simulink model "M009_refor_control_SOFC"  (R2021a)
settings: Solver=ode23tb  StartTime=0.0  StopTime=0.011794  RelTol=1e-3
undefined symbols (not defined in the file): MM_vec, nearst_p, p, Target, TotalMassTarget, Tr, Ts, x0_SOFC
libraries: pid_lib x1
settings Model: Creator=djoroya  LastModifiedBy=djoroya

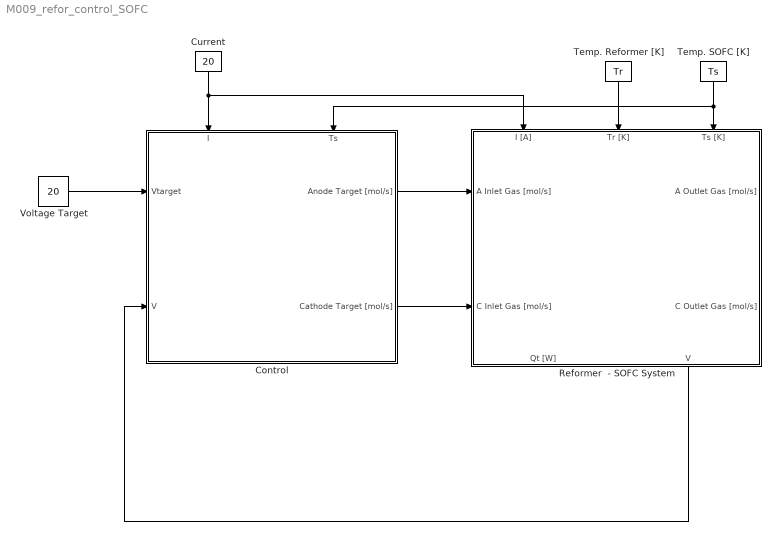
== system M009_refor_control_SOFC ==
  Control : Subsystem
      settings: PortSchema="{\"entries\":[{\"content\":{\"sides\":[{\"content\":{\"connectorIds\":[\"In1\",\"In2\"]},\"type\":\"ConnectorPlacement.EquallySpacedRectSide\",\"uuid\":\"b973b84c-8793-4046-ac9f-d89f915fcc30\"},{\"content\":{\"connectorIds\":[\"Out1\",\"Out2\"],\"side\":\"RIGHT\"},\"type\":\"ConnectorPlacement.EquallySpacedRectSide\",\"uuid\":\"99065125-60e5-4151-bf81-1bc55728c1bd\"},{\"content\":{\"connectorIds\":[\"In3\",\"In4\"],\"side\":\"TOP\"},\"type\":\"ConnectorPlacement.EquallySpacedRectSide\",\"uuid\":\"8b4e6a96-1b8a-4203-9bc5-ee7dbc8914e0\"}]},\"type\":\"ConnectorPlacement.EquallySpacedConnector\",\"uuid\":\"b75553d6-16dc-45b9-a76a-e219211962db\"}],\"packageUris\":[\"http://schema.mathworks.com/mf0/Connector/R2020b\"],\"version\":\"1.0\"}"
  Current : Constant  Value=20
  Reformer  - SOFC System : Subsystem
      settings: PortSchema="{\"entries\":[{\"content\":{\"sides\":[{\"content\":{\"connectorIds\":[\"In1\",\"In2\"]},\"type\":\"ConnectorPlacement.EquallySpacedRectSide\",\"uuid\":\"200e76d3-d0bd-400d-80aa-1287817324e9\"},{\"content\":{\"connectorIds\":[\"Out1\",\"Out2\"],\"side\":\"RIGHT\"},\"type\":\"ConnectorPlacement.EquallySpacedRectSide\",\"uuid\":\"3a1b6d1c-88bc-44b4-af37-27ac9ade1ff0\"},{\"content\":{\"connectorIds\":[\"In3\",\"In4\",\"In5\"],\"side\":\"TOP\"},\"type\":\"ConnectorPlacement.EquallySpacedRectSide\",\"uuid\":\"7d8c75f4-d537-4a2f-8caa-a1e3e4142219\"},{\"content\":{\"connectorIds\":[\"Out3\",\"Out4\"],\"side\":\"BOTTOM\"},\"type\":\"ConnectorPlacement.EquallySpacedRectSide\",\"uuid\":\"773ed184-9145-4e58-8690-ed7d817bf4e6\"}]},\"type\":\"ConnectorPlacement.EquallySpacedConnector\",\"uuid\":\"9e56a9e7-d63f-4491-bdfd-789be4cca736\"}],\"packageUris\":[\"http://schema.mathworks.com/mf0/Connector/R2020b\"],\"version\":\"1.0\"}"
  Temp. Reformer [K] : Constant  Value=Tr
  Temp. SOFC [K] : Constant  Value=Ts
  Voltage Target : Constant  Value=20
  wires:
  Control/1(Anode Target [mol/s]) -> Reformer  - SOFC System/1(A Inlet Gas [mol/s])
  Temp. Reformer [K]/1 -> Reformer  - SOFC System/4(Tr [K])
  Temp. SOFC [K]/1 -> Control/4(Ts), Reformer  - SOFC System/5(Ts [K])
  Control/2("Cathode Target [mol/s] ") -> Reformer  - SOFC System/2(C Inlet Gas [mol/s])
  Current/1 -> Reformer  - SOFC System/3(I [A]), Control/3(I)
  Voltage Target/1 -> Control/1(Vtarget)
  Reformer  - SOFC System/4(V) -> Control/2(V)

== system M009_refor_control_SOFC/Control ==
  Vtarget : Inport
  V : Inport  Port=2
  I : Inport  Port=3
  Ts : Inport  Port=4
  From Workspace : FromWorkspace  VariableName=air_mol_inlet_flow
  Product : Product
  Scope : Scope
  Target : Constant  Value=TotalMassTarget
  Target1 : Constant  Value=Target
  Anode Target [mol/s] : Outport
  "Cathode Target [mol/s] " : Outport  Port=2
  wires:
  From Workspace/1 -> "Cathode Target [mol/s] "/1
  Target/1 -> Product/2
  Product/1 -> Scope/1, Anode Target [mol/s]/1
  Target1/1 -> Product/1

== system M009_refor_control_SOFC/Reformer  - SOFC System ==
  note: Fuel
      | A node
      | (H2,O2,H2O,N2,CO,CH4,CO2,Diesel,Ar,Csoot)
      | [mol/s]
  A Inlet Gas [mol/s] : Inport
  C Inlet Gas [mol/s] : Inport  Port=2
  I [A] : Inport  Port=3
  Tr [K] : Inport  Port=4
  Ts [K] : Inport  Port=5
  Minus : Sum  Inputs=+-
  Product1 : Product
  Reformer Controlled : Subsystem
      settings: PortSchema="{\"entries\":[{\"content\":{\"sides\":[{\"content\":{\"connectorIds\":[\"In1\"]},\"type\":\"ConnectorPlacement.EquallySpacedRectSide\",\"uuid\":\"29baeb98-2fcd-4e93-bac7-89db238943a7\"},{\"content\":{\"connectorIds\":[\"Out1\"],\"side\":\"RIGHT\"},\"type\":\"ConnectorPlacement.EquallySpacedRectSide\",\"uuid\":\"d0aab1a2-46f5-4965-965a-81b00350cf0c\"},{\"content\":{\"connectorIds\":[\"In2\"],\"side\":\"TOP\"},\"type\":\"ConnectorPlacement.EquallySpacedRectSide\",\"uuid\":\"1acf7f26-ad42-41c1-b7e9-1e1e0c97fb8d\"}]},\"type\":\"ConnectorPlacement.EquallySpacedConnector\",\"uuid\":\"b24af2ad-4c30-4b70-9d7f-38f68bce100c\"}],\"packageUris\":[\"http://schema.mathworks.com/mf0/Connector/R2020b\"],\"version\":\"1.0\"}"
  SOFC Cell : Subsystem  mask{p=p, x0=x0_SOFC}
      mask prompts: p "params"
      settings: PortSchema="{\"entries\":[{\"content\":{\"sides\":[{\"content\":{\"connectorIds\":[\"In1\",\"In2\",\"In3\"]},\"type\":\"ConnectorPlacement.EquallySpacedRectSide\",\"uuid\":\"6cca8e4f-6db2-48de-a60a-b6fbc16877c6\"},{\"content\":{\"connectorIds\":[\"Out1\",\"Out2\",\"Out3\",\"Out4\"],\"side\":\"RIGHT\"},\"type\":\"ConnectorPlacement.EquallySpacedRectSide\",\"uuid\":\"c481f6d1-531d-4215-9ae0-5807376c0625\"},{\"content\":{\"connectorIds\":[\"In4\"],\"side\":\"TOP\"},\"type\":\"ConnectorPlacement.EquallySpacedRectSide\",\"uuid\":\"76720726-927e-4340-b17d-e33f4db2c782\"},{\"content\":{\"connectorIds\":[\"Out5\",\"Out6\"],\"side\":\"BOTTOM\"},\"type\":\"ConnectorPlacement.EquallySpacedRectSide\",\"uuid\":\"7ed108e3-6588-44d6-8f3d-9789ffe258a7\"}]},\"type\":\"ConnectorPlacement.EquallySpacedConnector\",\"uuid\":\"f9228f26-0840-43d6-932a-2fdb8a27bf20\"}],\"packageUris\":[\"http://schema.mathworks.com/mf0/Connector/R2020b\"],\"version\":\"1.0\"}"
  A Outlet Gas [mol/s] : Outport
  C Outlet Gas [mol/s] : Outport  Port=2
  Qt [W] : Outport  Port=3
  V : Outport  Port=4
  wires:
  A Inlet Gas [mol/s]/1 -> Reformer Controlled/1(Target MolarFlow [mol/s])
  SOFC Cell/5(EThermal) -> Minus/1  "ET"
  SOFC Cell/3(vc) -> C Outlet Gas [mol/s]/1  "pc_out [mol/s]"
  I [A]/1 -> SOFC Cell/2(I), Product1/2  "I"
  C Inlet Gas [mol/s]/1 -> SOFC Cell/3(Air[mol/s])
  SOFC Cell/6(Voltaje) -> Minus/2, V/1  "V"
  SOFC Cell/2(va) -> A Outlet Gas [mol/s]/1  "pa_out [mol/s]"
  Reformer Controlled/1(Actual Molar Flow [mol/s]) -> SOFC Cell/1(qin_anode)  "qin_anode"
  Product1/1 -> Qt [W]/1
  Minus/1 -> Product1/1
  Tr [K]/1 -> Reformer Controlled/2(T)
  Ts [K]/1 -> SOFC Cell/4(T)

== system M009_refor_control_SOFC/Reformer  - SOFC System/Reformer Controlled ==
  Target MolarFlow [mol/s] : Inport
  T : Inport  Port=2
  "Controler " : Subsystem
      settings: PortSchema="{\"entries\":[{\"content\":{\"sides\":[{\"content\":{\"connectorIds\":[\"In1\",\"In2\"]},\"type\":\"ConnectorPlacement.EquallySpacedRectSide\",\"uuid\":\"d0df8d63-6ccb-4e17-b5ac-849eda0159c4\"},{\"content\":{\"connectorIds\":[\"Out1\",\"Out2\",\"Out3\"],\"side\":\"RIGHT\"},\"type\":\"ConnectorPlacement.EquallySpacedRectSide\",\"uuid\":\"810d19ce-f80f-4df6-8135-9424920dd639\"},{\"content\":{\"connectorIds\":[],\"side\":\"TOP\"},\"type\":\"ConnectorPlacement.EquallySpacedRectSide\",\"uuid\":\"28b6769f-9191-4787-8749-9b059fcc021d\"},{\"content\":{\"connectorIds\":[\"In3\"],\"side\":\"BOTTOM\"},\"type\":\"ConnectorPlacement.EquallySpacedRectSide\",\"uuid\":\"5627e3a9-abda-41c8-96fd-097f9bf3cc2c\"}]},\"type\":\"ConnectorPlacement.EquallySpacedConnector\",\"uuid\":\"98d8d06d-7f78-4370-9651-63955ba4785e\"}],\"packageUris\":[\"http://schema.mathworks.com/mf0/Connector/R2020b\"],\"version\":\"1.0\"}"
  Gain : Gain  Gain=1./MM_vec
  Gain1 : Gain  Gain=MM_vec
  "Reformer " : Subsystem
  Actual Molar Flow [mol/s] : Outport
  wires:
  Gain/1 -> Actual Molar Flow [mol/s]/1  "out"
  Target MolarFlow [mol/s]/1 -> Gain1/1
  "Controler "/3(Steam) -> "Reformer "/3(Steam)  "Steam"
  "Controler "/2(Air) -> "Reformer "/2(Air)  "Air"
  "Controler "/1(Diesel) -> "Reformer "/1(Diesel)  "Diesel"
  Gain1/1 -> "Controler "/2(Target)
  T/1 -> "Controler "/3(T), "Reformer "/4(T)
  "Reformer "/1(MassFlows) -> "Controler "/1(MassFlow), Gain/1

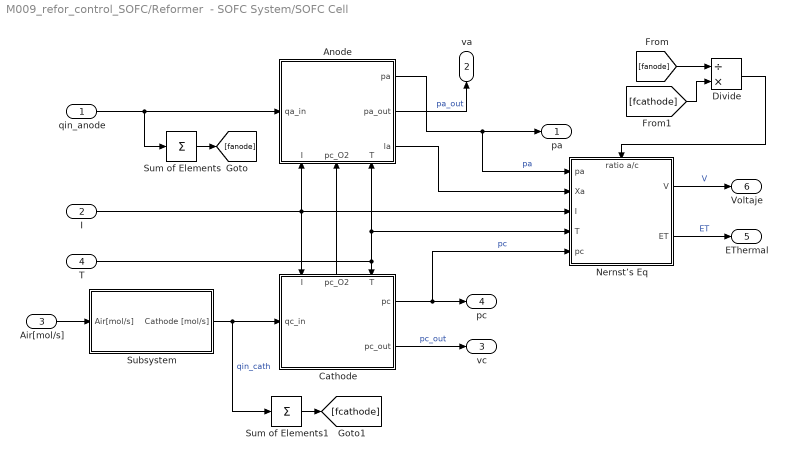
== system M009_refor_control_SOFC/Reformer  - SOFC System/SOFC Cell ==
  qin_anode : Inport
  I : Inport  Port=2
  Air[mol/s] : Inport  Port=3
  T : Inport  Port=4
  Anode : Subsystem
      settings: PortSchema="{\"entries\":[{\"content\":{\"sides\":[{\"content\":{\"connectorIds\":[\"In1\"]},\"type\":\"ConnectorPlacement.EquallySpacedRectSide\",\"uuid\":\"1d27f661-9cb9-482d-ac43-89e84d52643b\"},{\"content\":{\"connectorIds\":[\"Out1\",\"Out2\",\"Out3\"],\"side\":\"RIGHT\"},\"type\":\"ConnectorPlacement.EquallySpacedRectSide\",\"uuid\":\"62ac897d-5819-4e9c-a19f-e210851aefa2\"},{\"content\":{\"connectorIds\":[],\"side\":\"TOP\"},\"type\":\"ConnectorPlacement.EquallySpacedRectSide\",\"uuid\":\"1380e9d4-c5ac-42ce-b6fc-00336cc8edba\"},{\"content\":{\"connectorIds\":[\"In2\",\"In3\",\"In4\"],\"side\":\"BOTTOM\"},\"type\":\"ConnectorPlacement.EquallySpacedRectSide\",\"uuid\":\"0e36fd1a-38eb-48cb-8834-06d558b43614\"}]},\"type\":\"ConnectorPlacement.EquallySpacedConnector\",\"uuid\":\"79a72313-dbdc-4de5-b88f-787bafe984c7\"}],\"packageUris\":[\"http://schema.mathworks.com/mf0/Connector/R2020b\"],\"version\":\"1.0\"}"
  Cathode : Subsystem
      settings: PortSchema="{\"entries\":[{\"content\":{\"sides\":[{\"content\":{\"connectorIds\":[\"In1\"]},\"type\":\"ConnectorPlacement.EquallySpacedRectSide\",\"uuid\":\"1d27f661-9cb9-482d-ac43-89e84d52643b\"},{\"content\":{\"connectorIds\":[\"Out1\",\"Out2\"],\"side\":\"RIGHT\"},\"type\":\"ConnectorPlacement.EquallySpacedRectSide\",\"uuid\":\"62ac897d-5819-4e9c-a19f-e210851aefa2\"},{\"content\":{\"connectorIds\":[\"In2\",\"Out3\",\"In3\"],\"side\":\"TOP\"},\"type\":\"ConnectorPlacement.EquallySpacedRectSide\",\"uuid\":\"1380e9d4-c5ac-42ce-b6fc-00336cc8edba\"}]},\"type\":\"ConnectorPlacement.EquallySpacedConnector\",\"uuid\":\"79a72313-dbdc-4de5-b88f-787bafe984c7\"}],\"packageUris\":[\"http://schema.mathworks.com/mf0/Connector/R2020b\"],\"version\":\"1.0\"}"
  Divide : Product  Inputs=/*
  "Nernst’s Eq " : Subsystem
      settings: PortSchema="{\"entries\":[{\"content\":{\"sides\":[{\"content\":{\"connectorIds\":[\"In1\",\"In2\",\"In3\",\"In4\",\"In5\"]},\"type\":\"ConnectorPlacement.EquallySpacedRectSide\",\"uuid\":\"1b300774-e64d-4a8a-a2e9-ecdc71723fee\"},{\"content\":{\"connectorIds\":[\"Out1\",\"Out2\"],\"side\":\"RIGHT\"},\"type\":\"ConnectorPlacement.EquallySpacedRectSide\",\"uuid\":\"354a04f1-cc66-4a63-8c50-8080316e29e9\"},{\"content\":{\"connectorIds\":[\"In6\"],\"side\":\"TOP\"},\"type\":\"ConnectorPlacement.EquallySpacedRectSide\",\"uuid\":\"b48b7bda-dd37-468f-ab7d-ccd563a69f0b\"}]},\"type\":\"ConnectorPlacement.EquallySpacedConnector\",\"uuid\":\"ddfd4041-6e53-4893-9028-34e5ff9f82d6\"}],\"packageUris\":[\"http://schema.mathworks.com/mf0/Connector/R2020b\"],\"version\":\"1.0\"}"
  Subsystem : Subsystem
  Sum of Elements : Sum  Inputs=+
  Sum of Elements1 : Sum  Inputs=+
  pa : Outport
  va : Outport  Port=2
  vc : Outport  Port=3
  pc : Outport  Port=4
  EThermal : Outport  Port=5
  Voltaje : Outport  Port=6
  wires:
  Air[mol/s]/1 -> Subsystem/1(Air[mol/s])
  Anode/1(pa) -> pa/1, "Nernst’s Eq "/1(pa)  "pa"
  Anode/2(pa_out) -> va/1  "pa_out"
  Cathode/1(pc) -> "Nernst’s Eq "/5(pc), pc/1  "pc"
  Subsystem/1(Cathode [mol/s]) -> Sum of Elements1/1, Cathode/1(qc_in)  "qin_cath"
  "Nernst’s Eq "/2(ET) -> EThermal/1  "ET"
  Cathode/3(pc_O2) -> Anode/3(pc_O2)
  Cathode/2(pc_out) -> vc/1  "pc_out"
  I/1 -> Cathode/2(I), "Nernst’s Eq "/3(I), Anode/2(I)
  T/1 -> "Nernst’s Eq "/4(T), Anode/4(T), Cathode/3(T)
  qin_anode/1 -> Anode/1(qa_in), Sum of Elements/1
  "Nernst’s Eq "/1(V) -> Voltaje/1  "V"
  Anode/3(la) -> "Nernst’s Eq "/2(Xa)
  Sum of Elements/1 -> [fanode]
  Sum of Elements1/1 -> [fcathode]
  [fanode] -> Divide/1
  [fcathode] -> Divide/2
  Divide/1 -> "Nernst’s Eq "/6(ratio a/c)

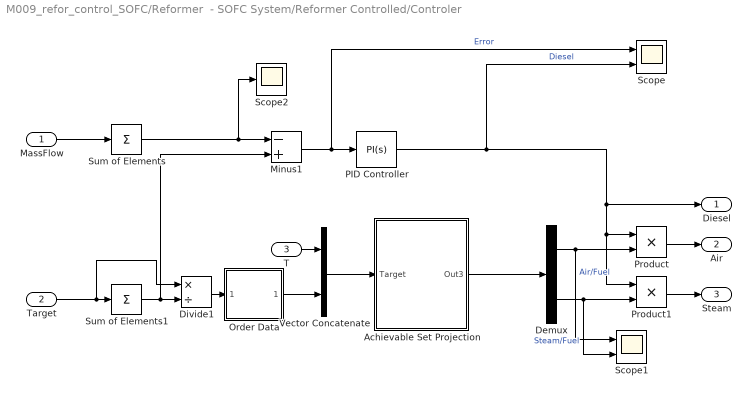
== system M009_refor_control_SOFC/Reformer  - SOFC System/Reformer Controlled/Controler  ==
  MassFlow : Inport
  Target : Inport  Port=2
  T : Inport  Port=3
  Achievable Set Projection : Subsystem
  Demux : Demux  Outputs=2
  Divide1 : Product  Inputs=*/
  Minus1 : Sum  Inputs=-+
  Order Data : Subsystem
  PID Controller : pid_lib/PID Controller  Controller=PI  Form=Parallel  TimeDomain=Continuous-time  UseExternalTs=off  SampleTime=-1  IntegratorMethod=Forward Euler  FilterMethod=Forward Euler  ControllerParametersSource=internal  P=10  I=50  D=1  UseFilter=on  N=100  TunerSelectOption=Transfer Function Based (PID Tuner App)  ZeroCross=off  InitialConditionSource=internal  InitialConditionForIntegrator=0  InitialConditionForFilter=0  DifferentiatorICPrevScaledInput=0  ExternalReset=none  TrackingMode=off  Kt=1  LimitOutput=off  SatLimitsSource=internal  UpperSaturationLimit=inf  LowerSaturationLimit=-inf  LinearizeAsGain=on  AntiWindupMode=none  Kb=1  POutMin=[]  POutMax=[]  IOutMin=[]  IOutMax=[]  DOutMin=[]  DOutMax=[]  NOutMin=[]  NOutMax=[]  SumOutMin=[]  SumOutMax=[]  SaturationOutMin=[]  SaturationOutMax=[]  PParamMin=[]  PParamMax=[]  IParamMin=[]  IParamMax=[]  DParamMin=[]  DParamMax=[]  NParamMin=[]  NParamMax=[]  KbParamMin=[]  KbParamMax=[]  KtParamMin=[]  KtParamMax=[]  KbOutMin=[]  KbOutMax=[]  KtOutMin=[]  KtOutMax=[]  IntegratorOutMin=[]  IntegratorOutMax=[]  FilterOutMin=[]  FilterOutMax=[]  SumI1OutMin=[]  SumI1OutMax=[]  SumI2OutMin=[]  SumI2OutMax=[]  SumI3OutMin=[]  SumI3OutMax=[]  SumI4OutMin=[]  SumI4OutMax=[]  SumDOutMin=[]  SumDOutMax=[]  DifferentiatorOutMin=[]  DifferentiatorOutMax=[]  FilterDiffOutCoefMin=[]  FilterDiffOutCoefMax=[]  ReciprocalOutMin=[]  ReciprocalOutMax=[]  SumDenOutMin=[]  SumDenOutMax=[]  SumNumOutMin=[]  SumNumOutMax=[]  DivideOutMin=[]  DivideOutMax=[]  UdiffTsProdOutMin=[]  UdiffTsProdOutMax=[]  NTsProdOutMin=[]  NTsProdOutMax=[]  UintegralTsProdOutMin=[]  UintegralTsProdOutMax=[]  UngainTsProdOutMin=[]  UngainTsProdOutMax=[]  IntegratorContinuousStateAttributes=''  IntegratorStateMustResolveToSignalObject=off  IntegratorRTWStateStorageClass=Auto  FilterContinuousStateAttributes=''  FilterStateMustResolveToSignalObject=off  FilterRTWStateStorageClass=Auto  ParallelPVariant=InternalParameters  IdealPVariant=Disabled  IVariant=InternalParameters  DVariant=Disabled  IntegratorVariant=Continuous  SatVariant=Disabled  AWVariant=Passthrough  PCopyVariant=Disabled  TRVariant=Disabled  FdbkBlocksVariant=Forward  IdealPFdbkVariant=Disabled  SatFdbkVariant=Disabled  DerivativeFilterVariant=Disabled  NVariant=Disabled  NCopyVariant=Disabled_SignalSpec  FilterICVariant=Disabled  IntegratorICVariant=InternalICs  ExternalResetVariant=Disabled  TRSumVariant=Passthrough  SumFdbkVariant=Disabled  SumVariant=Sum_PI  TsampFilterVariant=InternalTs  TsampNgainVariant=Passthrough  TsampIntegralVariant=Passthrough  ExternalSaturationOutDataTypeStr=Inherit: Same as second input
  Product : Product
  Product1 : Product
  Scope : Scope  NumInputPorts=2
  Scope1 : Scope  NumInputPorts=2
  Scope2 : Scope
  Sum of Elements : Sum  Inputs=+
  Sum of Elements1 : Sum  Inputs=+
  Vector Concatenate : Concatenate
  Diesel : Outport
  Air : Outport  Port=2
  Steam : Outport  Port=3
  wires:
  Product/1 -> Air/1
  Demux/1 -> Scope1/1, Product/2  "Air/Fuel"
  Demux/2 -> Scope1/2, Product1/2  "Steam/Fuel"
  Product1/1 -> Steam/1
  Sum of Elements/1 -> Scope2/1, Minus1/1
  T/1 -> Vector Concatenate/1
  Order Data/1(Out1) -> Vector Concatenate/2
  Sum of Elements1/1 -> Divide1/2, Minus1/2
  Target/1 -> Divide1/1, Sum of Elements1/1
  Divide1/1 -> Order Data/1(Target)
  Minus1/1 -> PID Controller/1, Scope/1  "Error"
  MassFlow/1 -> Sum of Elements/1
  PID Controller/1 -> Product1/1, Product/1, Diesel/1, Scope/2  "Diesel"
  Vector Concatenate/1 -> Achievable Set Projection/1(Target)
  Achievable Set Projection/1(Out3) -> Demux/1

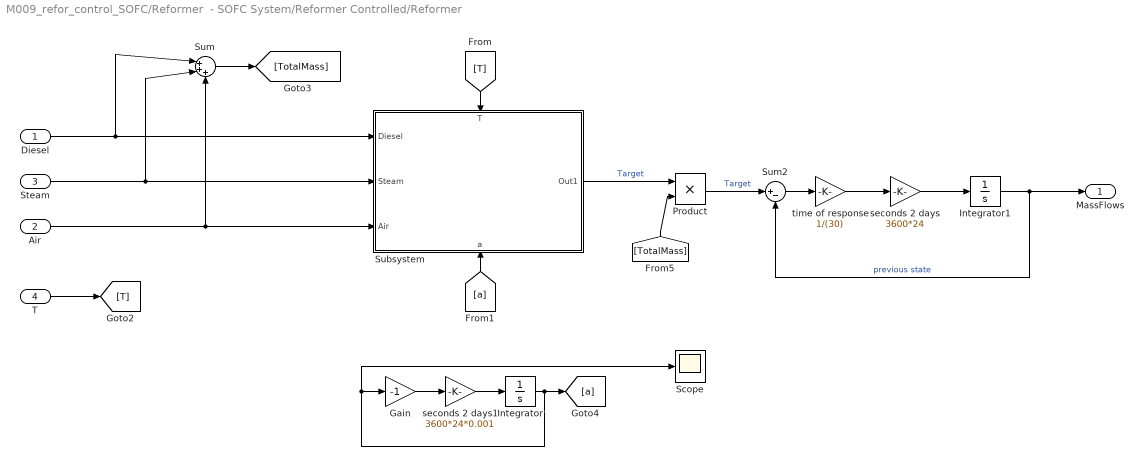
== system M009_refor_control_SOFC/Reformer  - SOFC System/Reformer Controlled/Reformer  ==
  Diesel : Inport
  Air : Inport  Port=2
  Steam : Inport  Port=3
  T : Inport  Port=4
  Gain : Gain  Gain=-1
  Integrator : Integrator  InitialCondition=1
  Integrator1 : Integrator  InitialCondition=1e-6
  Product : Product
  Scope : Scope
  Subsystem : Subsystem
      settings: PortSchema="{\"entries\":[{\"content\":{\"sides\":[{\"content\":{\"connectorIds\":[\"In1\",\"In2\",\"In3\"]},\"type\":\"ConnectorPlacement.EquallySpacedRectSide\",\"uuid\":\"0dada652-6957-4c3e-8e48-73ee360a3bab\"},{\"content\":{\"connectorIds\":[\"Out1\"],\"side\":\"RIGHT\"},\"type\":\"ConnectorPlacement.EquallySpacedRectSide\",\"uuid\":\"81208621-951c-43f9-b655-3502a16ce57a\"},{\"content\":{\"connectorIds\":[\"In4\"],\"side\":\"TOP\"},\"type\":\"ConnectorPlacement.EquallySpacedRectSide\",\"uuid\":\"1012e2be-7d0b-44a9-9a40-bc453950010e\"},{\"content\":{\"connectorIds\":[\"In5\"],\"side\":\"BOTTOM\"},\"type\":\"ConnectorPlacement.EquallySpacedRectSide\",\"uuid\":\"aaef83a2-abb7-4780-82b5-9abad57d39ad\"}]},\"type\":\"ConnectorPlacement.EquallySpacedConnector\",\"uuid\":\"1143871f-aacc-4fa7-a444-9910d5016eff\"}],\"packageUris\":[\"http://schema.mathworks.com/mf0/Connector/R2020b\"],\"version\":\"1.0\"}"
  Sum : Sum  Inputs=|+++
  Sum2 : Sum  Inputs=|+-
  seconds 2 days : Gain  Gain=3600*24
  seconds 2 days1 : Gain  Gain=3600*24*0.001
  time of response : Gain  Gain=1/(30)
  MassFlows : Outport
  wires:
  T/1 -> [T]
  Sum/1 -> [TotalMass]
  [TotalMass] -> Product/2
  Diesel/1 -> Sum/1, Subsystem/1(Diesel)
  seconds 2 days1/1 -> Integrator/1
  Gain/1 -> seconds 2 days1/1
  [a] -> Subsystem/5(a)
  [T] -> Subsystem/4(T)
  time of response/1 -> seconds 2 days/1
  Sum2/1 -> time of response/1
  Product/1 -> Sum2/1  "Target"
  seconds 2 days/1 -> Integrator1/1
  Integrator1/1 -> MassFlows/1, Sum2/2  "previous state"
  Subsystem/1(Out1) -> Product/1  "Target"
  Steam/1 -> Sum/2, Subsystem/2(Steam)
  Air/1 -> Sum/3, Subsystem/3(Air)
  Integrator/1 -> Scope/1, Gain/1, [a]

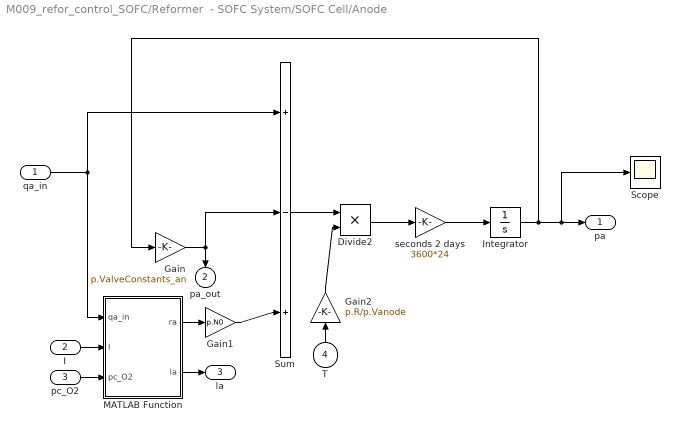
== system M009_refor_control_SOFC/Reformer  - SOFC System/SOFC Cell/Anode ==
  qa_in : Inport
  I : Inport  Port=2
  pc_O2 : Inport  Port=3
  T : Inport  Port=4
  Divide2 : Product  Inputs=**
  Gain : Gain  Gain=p.ValveConstants_an
  Gain1 : Gain  Gain=p.N0
  Gain2 : Gain  Gain=p.R/p.Vanode
  Integrator : Integrator  InitialCondition=x0_SOFC.pa
  MATLAB Function : MATLAB Function  TreatAsAtomicUnit=on
  Scope : Scope
  Sum : Sum  Inputs=|+-+
  seconds 2 days : Gain  Gain=3600*24
  pa : Outport
  pa_out : Outport  Port=2
  la : Outport  Port=3
  wires:
  Sum/1 -> Divide2/1
  Integrator/1 -> Scope/1, pa/1, Gain/1
  Gain2/1 -> Divide2/2
  qa_in/1 -> Sum/1, MATLAB Function/1(qa_in)
  Gain/1 -> pa_out/1, Sum/2
  I/1 -> MATLAB Function/2(I)
  T/1 -> Gain2/1
  MATLAB Function/2(la) -> la/1
  pc_O2/1 -> MATLAB Function/3(pc_O2)
  MATLAB Function/1(ra) -> Gain1/1
  Gain1/1 -> Sum/3
  Divide2/1 -> seconds 2 days/1
  seconds 2 days/1 -> Integrator/1

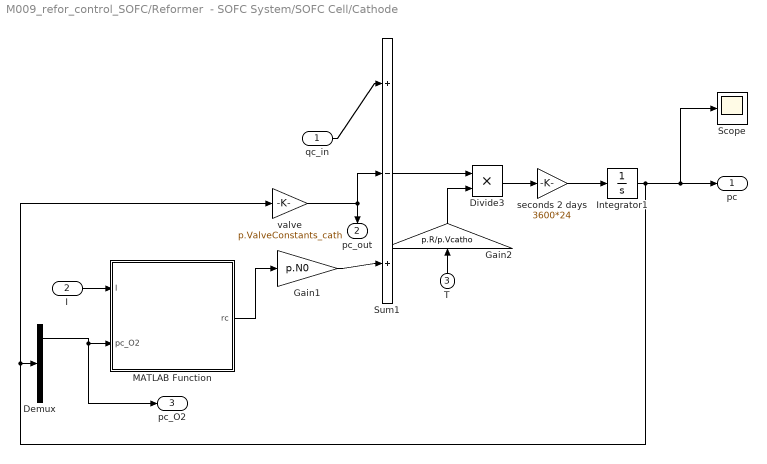
== system M009_refor_control_SOFC/Reformer  - SOFC System/SOFC Cell/Cathode ==
  qc_in : Inport
  I : Inport  Port=2
  T : Inport  Port=3
  Demux : Demux  Outputs=8
  Divide3 : Product  Inputs=**
  Gain1 : Gain  Gain=p.N0
  Gain2 : Gain  Gain=p.R/p.Vcatho
  Integrator1 : Integrator  InitialCondition=x0_SOFC.pc
  MATLAB Function : MATLAB Function  TreatAsAtomicUnit=on
  Scope : Scope
  Sum1 : Sum  Inputs=|+-+
  seconds 2 days : Gain  Gain=3600*24
  valve : Gain  Gain=p.ValveConstants_cath
  pc : Outport
  pc_out : Outport  Port=2  Unit=mol/s
  pc_O2 : Outport  Port=3
  wires:
  Sum1/1 -> Divide3/1
  Integrator1/1 -> valve/1, Demux/1, Scope/1, pc/1
  qc_in/1 -> Sum1/1
  Gain2/1 -> Divide3/2
  T/1 -> Gain2/1
  valve/1 -> pc_out/1, Sum1/2
  I/1 -> MATLAB Function/1(I)
  Demux/2 -> pc_O2/1, MATLAB Function/2(pc_O2)
  MATLAB Function/1(rc) -> Gain1/1
  Gain1/1 -> Sum1/3
  Divide3/1 -> seconds 2 days/1
  seconds 2 days/1 -> Integrator1/1

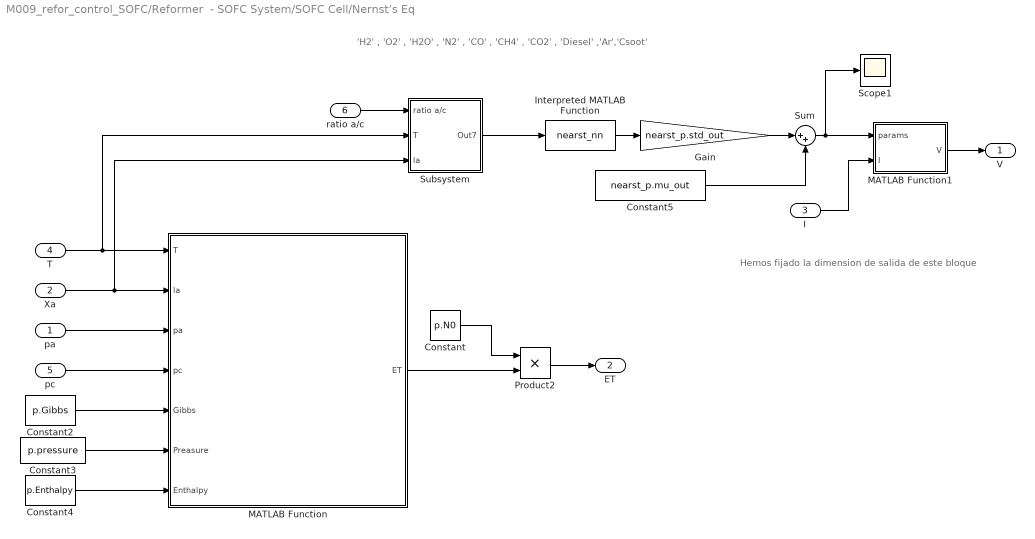
== system M009_refor_control_SOFC/Reformer  - SOFC System/SOFC Cell/Nernst’s Eq  ==
  note: Hemos fijado la dimension de salida de este bloque
  note: 'H2' , 'O2' , 'H2O' , 'N2' , 'CO' , 'CH4' , 'CO2' , 'Diesel' ,'Ar','Csoot'
  pa : Inport
  Xa : Inport  Port=2
  I : Inport  Port=3
  T : Inport  Port=4
  pc : Inport  Port=5
  ratio a/c : Inport  Port=6
  Constant : Constant  Value=p.N0
  Constant2 : Constant  Value=p.Gibbs  OutDataTypeStr=Bus:slBus1
  Constant3 : Constant  Value=p.pressure
  Constant4 : Constant  Value=p.Enthalpy  OutDataTypeStr=Bus:slBus1
  Constant5 : Constant  Value=nearst_p.mu_out
  Gain : Gain  Gain=nearst_p.std_out
  Interpreted MATLAB Function : MATLABFcn  MATLABFcn=nearst_nn
  MATLAB Function : MATLAB Function  TreatAsAtomicUnit=on
  MATLAB Function1 : MATLAB Function  TreatAsAtomicUnit=on
  Product2 : Product
  Scope1 : Scope
  Subsystem : Subsystem
  Sum : Sum  Inputs=|++
  V : Outport  PortDimensions=1
  ET : Outport  Port=2  PortDimensions=1
  wires:
  pa/1 -> MATLAB Function/3(pa)
  pc/1 -> MATLAB Function/4(pc)
  Constant2/1 -> MATLAB Function/5(Gibbs)
  T/1 -> MATLAB Function/1(T), Subsystem/2(T)
  Xa/1 -> MATLAB Function/2(la), Subsystem/3(la)
  Constant3/1 -> MATLAB Function/6(Preasure)
  Constant4/1 -> MATLAB Function/7(Enthalpy)
  Product2/1 -> ET/1
  MATLAB Function/1(ET) -> Product2/2
  ratio a/c/1 -> Subsystem/1(ratio a/c)
  Subsystem/1(Out7) -> Interpreted MATLAB Function/1
  Interpreted MATLAB Function/1 -> Gain/1
  Gain/1 -> Sum/1
  Constant5/1 -> Sum/2
  Sum/1 -> Scope1/1, MATLAB Function1/1(params)
  MATLAB Function1/1(V) -> V/1
  Constant/1 -> Product2/1
  I/1 -> MATLAB Function1/2(I)

== system M009_refor_control_SOFC/Reformer  - SOFC System/SOFC Cell/Subsystem ==
  Air[mol/s] : Inport
  Molar Fractions (H2,O2,H2O,N2,CO,CH4,CO2) [mol/(Air-mol)] : Constant  Value=[0 0.2095 0 0.7808 0 0 0 0 0 0]
  Product : Product
  Cathode [mol/s] : Outport
  wires:
  Air[mol/s]/1 -> Product/1  "Air [mol/s]"
  Product/1 -> Cathode [mol/s]/1  "Cathode [mol/s]"
  Molar Fractions (H2,O2,H2O,N2,CO,CH4,CO2) [mol/(Air-mol)]/1 -> Product/2

== system M009_refor_control_SOFC/Reformer  - SOFC System/Reformer Controlled/Controler /Achievable Set Projection ==
  Target : Inport
  Abs : Abs
  Equilibrium2Ratios : MATLABFcn  MATLABFcn=backward_reformer_net  OutputDimensions=2  OutputSignalType=real  Output1D=off
  If : If  IfExpression=u1 > 0.01
  If Action Subsystem : Subsystem  TreatAsAtomicUnit=on
  If Action Subsystem1 : Subsystem  TreatAsAtomicUnit=on
  Merge : Merge
  ¿Convex hull? : MATLABFcn  MATLABFcn=check_convex_hull  OutputDimensions=1  OutputSignalType=real  Output1D=off
  Out3 : Outport
  wires:
  ¿Convex hull?/1 -> If/1
  Target/1 -> If Action Subsystem1/1(Target), If Action Subsystem/1(Target), ¿Convex hull?/1
  If/1 -> If Action Subsystem/Action
  If/2 -> If Action Subsystem1/Action
  Merge/1 -> Equilibrium2Ratios/1
  If Action Subsystem/1(Out1) -> Merge/1
  If Action Subsystem1/1(Out1) -> Merge/2
  Equilibrium2Ratios/1 -> Abs/1
  Abs/1 -> Out3/1

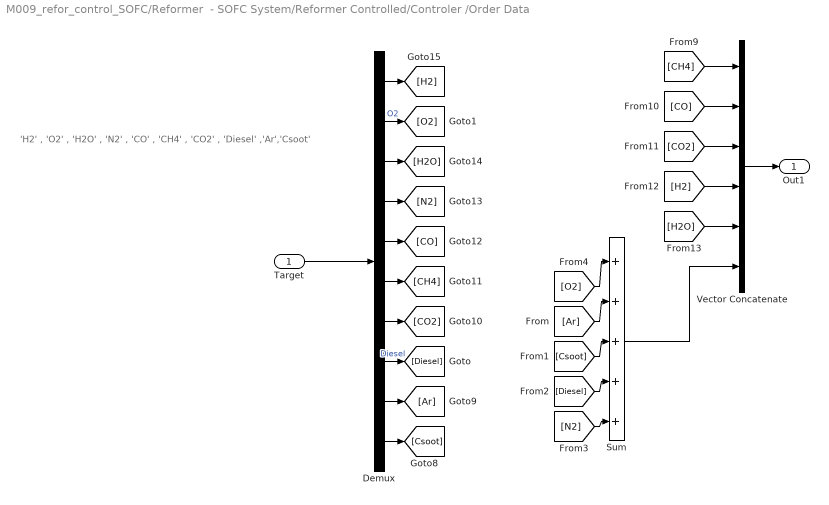
== system M009_refor_control_SOFC/Reformer  - SOFC System/Reformer Controlled/Controler /Order Data ==
  note: 'H2' , 'O2' , 'H2O' , 'N2' , 'CO' , 'CH4' , 'CO2' , 'Diesel' ,'Ar','Csoot'
  Target : Inport
  Demux : Demux  Outputs=10
  Sum : Sum  Inputs=|+++++
  Vector Concatenate : Concatenate  NumInputs=6
  Out1 : Outport
  wires:
  Target/1 -> Demux/1
  [CO] -> Vector Concatenate/2
  [CO2] -> Vector Concatenate/3
  [H2] -> Vector Concatenate/4
  [H2O] -> Vector Concatenate/5
  Vector Concatenate/1 -> Out1/1
  Demux/1 -> [H2]
  Demux/3 -> [H2O]
  Demux/4 -> [N2]
  Demux/5 -> [CO]
  Demux/6 -> [CH4]
  Demux/7 -> [CO2]
  Demux/9 -> [Ar]
  Demux/10 -> [Csoot]
  [CH4] -> Vector Concatenate/1
  Demux/2 -> [O2]  "O2"
  Demux/8 -> [Diesel]  "Diesel"
  [O2] -> Sum/1
  [Ar] -> Sum/2
  [Csoot] -> Sum/3
  [Diesel] -> Sum/4
  [N2] -> Sum/5
  Sum/1 -> Vector Concatenate/6

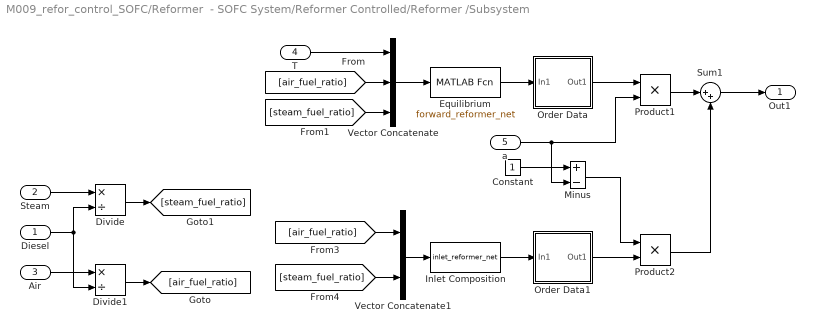
== system M009_refor_control_SOFC/Reformer  - SOFC System/Reformer Controlled/Reformer /Subsystem ==
  Diesel : Inport
  Steam : Inport  Port=2
  Air : Inport  Port=3
  T : Inport  Port=4
  a : Inport  Port=5
  Constant : Constant
  Divide : Product  Inputs=*/
  Divide1 : Product  Inputs=*/
  Equilibrium : MATLABFcn  MATLABFcn=forward_reformer_net  OutputDimensions=8  OutputSignalType=real  Output1D=off
  Inlet Composition : MATLABFcn  MATLABFcn=inlet_reformer_net  OutputDimensions=6  OutputSignalType=real  Output1D=off
  Minus : Sum  Inputs=+-
  Order Data : Subsystem
  Order Data1 : Subsystem
  Product1 : Product
  Product2 : Product
  Sum1 : Sum  Inputs=|++
  Vector Concatenate : Concatenate  NumInputs=3
  Vector Concatenate1 : Concatenate
  Out1 : Outport
  wires:
  a/1 -> Product1/2, Minus/2
  [steam_fuel_ratio] -> Vector Concatenate/3
  Product1/1 -> Sum1/1
  T/1 -> Vector Concatenate/1
  [air_fuel_ratio] -> Vector Concatenate1/1
  Vector Concatenate/1 -> Equilibrium/1
  Product2/1 -> Sum1/2
  [steam_fuel_ratio] -> Vector Concatenate1/2
  Order Data1/1(Out1) -> Product2/2
  Minus/1 -> Product2/1
  Inlet Composition/1 -> Order Data1/1(In1)
  Order Data/1(Out1) -> Product1/1
  Vector Concatenate1/1 -> Inlet Composition/1
  [air_fuel_ratio] -> Vector Concatenate/2
  Equilibrium/1 -> Order Data/1(In1)
  Constant/1 -> Minus/1
  Sum1/1 -> Out1/1
  Steam/1 -> Divide/1
  Diesel/1 -> Divide1/2, Divide/2
  Air/1 -> Divide1/1
  Divide/1 -> [steam_fuel_ratio]
  Divide1/1 -> [air_fuel_ratio]

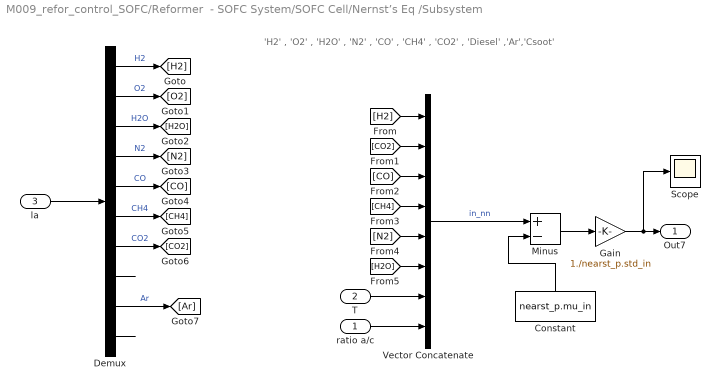
== system M009_refor_control_SOFC/Reformer  - SOFC System/SOFC Cell/Nernst’s Eq /Subsystem ==
  note: 'H2' , 'O2' , 'H2O' , 'N2' , 'CO' , 'CH4' , 'CO2' , 'Diesel' ,'Ar','Csoot'
  ratio a/c : Inport
  T : Inport  Port=2
  la : Inport  Port=3
  Constant : Constant  Value=nearst_p.mu_in
  Demux : Demux  Outputs=10
  Gain : Gain  Gain=1./nearst_p.std_in
  Minus : Sum  Inputs=+-
  Scope : Scope
  Vector Concatenate : Concatenate  NumInputs=8
  Out7 : Outport
  wires:
  Demux/7 -> [CO2]  "CO2"
  la/1 -> Demux/1
  Demux/3 -> [H2O]  "H2O"
  Demux/1 -> [H2]  "H2"
  Demux/8 -> ?
  Demux/2 -> [O2]  "O2"
  Demux/10 -> ?
  Demux/9 -> [Ar]  "Ar"
  Demux/5 -> [CO]  "CO"
  Demux/4 -> [N2]  "N2"
  Demux/6 -> [CH4]  "CH4"
  ratio a/c/1 -> Vector Concatenate/8
  T/1 -> Vector Concatenate/7
  [H2] -> Vector Concatenate/1
  [CO2] -> Vector Concatenate/2
  [CO] -> Vector Concatenate/3
  [CH4] -> Vector Concatenate/4
  [N2] -> Vector Concatenate/5
  [H2O] -> Vector Concatenate/6
  Vector Concatenate/1 -> Minus/1  "in_nn"
  Constant/1 -> Minus/2
  Minus/1 -> Gain/1
  Gain/1 -> Scope/1, Out7/1

== system M009_refor_control_SOFC/Reformer  - SOFC System/Reformer Controlled/Controler /Achievable Set Projection/If Action Subsystem ==
  Target : Inport
  Action Port : ActionPort  ActionPortLabel=if(u1 > 0.01)
  Demux : Demux  Outputs=7
  Vector Concatenate : Concatenate
  proyection : MATLABFcn  MATLABFcn=proyection_in_convex_hull  OutputDimensions=6  OutputSignalType=real  Output1D=off
  Out1 : Outport
  wires:
  Target/1 -> Demux/1, proyection/1
  proyection/1 -> Vector Concatenate/2
  Demux/1 -> Vector Concatenate/1
  Vector Concatenate/1 -> Out1/1

== system M009_refor_control_SOFC/Reformer  - SOFC System/Reformer Controlled/Controler /Achievable Set Projection/If Action Subsystem1 ==
  Target : Inport
  Action Port : ActionPort  ActionPortLabel=else
  Out1 : Outport
  wires:
  Target/1 -> Out1/1

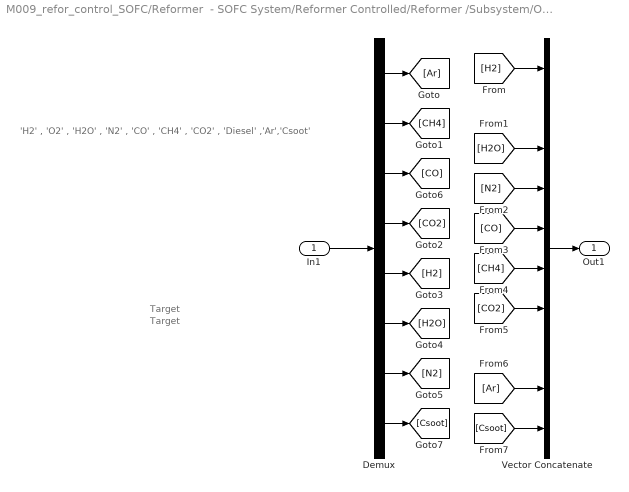
== system M009_refor_control_SOFC/Reformer  - SOFC System/Reformer Controlled/Reformer /Subsystem/Order Data ==
  note: Target
  note: Target
  note: 'H2' , 'O2' , 'H2O' , 'N2' , 'CO' , 'CH4' , 'CO2' , 'Diesel' ,'Ar','Csoot'
  In1 : Inport
  Demux : Demux  Outputs=8
  Vector Concatenate : Concatenate  NumInputs=10
  Out1 : Outport
  wires:
  In1/1 -> Demux/1
  Demux/1 -> [Ar]
  Demux/2 -> [CH4]
  Demux/3 -> [CO]
  Demux/4 -> [CO2]
  Demux/5 -> [H2]
  Demux/6 -> [H2O]
  Demux/7 -> [N2]
  Demux/8 -> [Csoot]
  [H2] -> Vector Concatenate/1
  [H2O] -> Vector Concatenate/3
  [N2] -> Vector Concatenate/4
  [CO] -> Vector Concatenate/5
  [CH4] -> Vector Concatenate/6
  [CO2] -> Vector Concatenate/7
  [Ar] -> Vector Concatenate/9
  [Csoot] -> Vector Concatenate/10
  Vector Concatenate/1 -> Out1/1

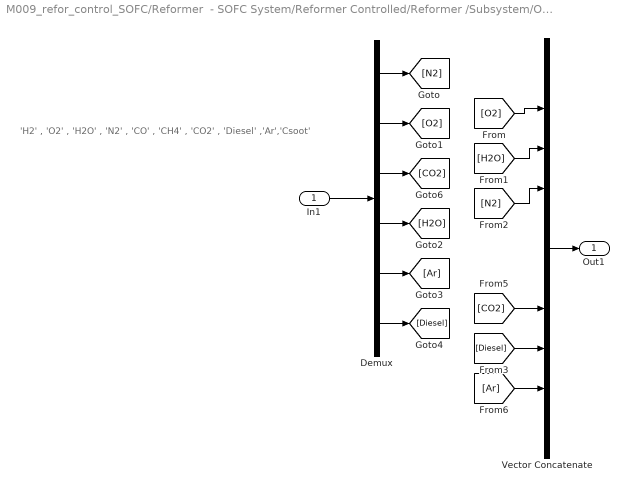
== system M009_refor_control_SOFC/Reformer  - SOFC System/Reformer Controlled/Reformer /Subsystem/Order Data1 ==
  note: 'H2' , 'O2' , 'H2O' , 'N2' , 'CO' , 'CH4' , 'CO2' , 'Diesel' ,'Ar','Csoot'
  In1 : Inport
  Demux : Demux  Outputs=6
  Vector Concatenate : Concatenate  NumInputs=10
  Out1 : Outport
  wires:
  In1/1 -> Demux/1
  Demux/1 -> [N2]
  Demux/2 -> [O2]
  Demux/3 -> [CO2]
  Demux/4 -> [H2O]
  Demux/5 -> [Ar]
  Demux/6 -> [Diesel]
  [H2O] -> Vector Concatenate/3
  [N2] -> Vector Concatenate/4
  [CO2] -> Vector Concatenate/7
  [Ar] -> Vector Concatenate/9
  Vector Concatenate/1 -> Out1/1
  [O2] -> Vector Concatenate/2
  [Diesel] -> Vector Concatenate/8

== matlab function M009_refor_control_SOFC/Reformer  - SOFC System/SOFC Cell/Cathode/MATLAB Function ==
  data: rc output; I input; pc_O2 input
function rc = fcn(I,pc_O2)

%l = qc_in/sum(qc_in);

% l_H2  = l(1);
% l_O2  = l(2);
% l_H2O = l(3);
% l_N2  = l(4);
% l_CO  = l(5);
% l_CH4 = l(6);
% l_CO2 = l(7);
%
% alpha_H_2 = l_H2;
% alpha_CO  = l_CO;
% alpha_CH4 = l_CH4;
% alpha_O2  = 0.5*(l_H2+l_CO+4*l_CH4);
% beta_H2O  = l_H2 + 2*l_CH4;
% beta_CO2  = l_CO + 2*l_CH4;
%
F = 96485.3329; 

% r_H2  = -alpha_H_2*I;
% r_CO  = -alpha_CO*I;
% r_CH4 = -alpha_CH4*I;
% r_H20 = beta_H2O*I;
% r_CO2 = beta_CO2*I;
if pc_O2 <= 0
    r_O2  = 0;
else
    r_O2  = I/(4*F);
end

rc = [0 -r_O2 0 0 0 0 0 0 0 0]';

== matlab function M009_refor_control_SOFC/Reformer  - SOFC System/SOFC Cell/Anode/MATLAB Function ==
  data: qa_in input; ra output; I input; la output; pc_O2 input
function [ra,la] = fcn(qa_in,I,pc_O2)

la = qa_in/sum(qa_in);

l_H2  = la(1);
%l_O2  = l(2);
%l_H2O = l(3);
%l_N2  = l(4);
l_CO  = la(5);
l_CH4 = la(6);
%l_CO2 = l(7);
%
alpha_H2 = l_H2;
alpha_CO  = l_CO;
alpha_CH4 = l_CH4;
%alpha_O2  = 0.5*(l_H2+l_CO+4*l_CH4);
beta_H2O  = l_H2 + 2*l_CH4;
beta_CO2  = l_CO + l_CH4;
%
F = 96485.3329; 
ne = 2*(l_H2 + l_CO + 4*l_CH4);
I = I/(F*ne);

r_H2  = -alpha_H2*I;
r_CO  = -alpha_CO*I;
r_CH4 = -alpha_CH4*I;
r_H20 = beta_H2O*I;
r_CO2 = beta_CO2*I;
%
ra = [r_H2 0 r_H20 0 r_CO r_CH4 r_CO2 0 0 0]';

if pc_O2 <= 0
    ra  = 0*ra;
end

== matlab function M009_refor_control_SOFC/Reformer  - SOFC System/SOFC Cell/Nernst’s Eq /MATLAB Function ==
  data: T input; la input; pa input; pc input; Gibbs input; Preasure input; Enthalpy input; ET output
function ET  = fcn(T, la,pa,pc,Gibbs,Preasure, Enthalpy)
%

l_H2  = la(1);
l_CO  = la(5);
l_CH4 = la(6);
%
alpha_H2 = l_H2;
alpha_CO  = l_CO;
alpha_CH4 = l_CH4;
alpha_O2  = 0.5*( l_H2 + l_CO + 4*l_CH4);
beta_H2O  = l_H2 + 2*l_CH4;
beta_CO2  = l_CO + l_CH4;

%
pa_H2 = pa(1);
pa_O2 = pa(2);
pa_H2O= pa(3);
pa_CO = pa(5);
pa_CH4= pa(6);
pa_CO2= pa(7);
%
pc_H2 = pc(1);
pc_O2 = pc(2);
pc_H2O= pc(3);
pc_N2 = pc(4);
pc_CO = pc(5);
pc_CH4= pc(6);
pc_CO2= pc(7);
%% 
F = 96485.3329; 
ne = 2*(l_H2 + l_CO + 4*l_CH4);
%%
G = alpha_H2*Gibbs.H2 + ...
    alpha_CO*Gibbs.CO + ...
    alpha_CH4*Gibbs.CH4 + ...
    alpha_O2*Gibbs.O2 + ...
    - beta_H2O*Gibbs.H2O + ...
    - beta_CO2*Gibbs.CO2;
%%
E0 = G/(F*ne); 

%%
R = 8.31446261815324;

ab =    [alpha_H2, ...
         alpha_CO, ...
         alpha_CH4, ...
         alpha_O2,  ...
         -beta_H2O, ...
         -beta_CO2];
     
pa_ab = [pa_H2, ...
         pa_CO, ...
         pa_CH4, ...
         pc_O2,  ...
         pa_H2O, ...
         pa_CO2];
     
log_ab = 0*ab;
iter = 0;
for ipa_ab = pa_ab
    iter = iter + 1;
    if ipa_ab > 0
       log_ab(iter) =  log(ipa_ab/Preasure);
    end
end

E = E0 + ((R*T)/(ne*F))*( sum(log_ab.*ab) );

%%
H = alpha_H2*Enthalpy.H2 + ...
    alpha_CO*Enthalpy.CO + ...
    alpha_CH4*Enthalpy.CH4 + ...
    alpha_O2*Enthalpy.O2 + ...
    - beta_H2O*Enthalpy.H2O + ...
    - beta_CO2*Enthalpy.CO2;
ET = H/(ne*F);
%

== matlab function M009_refor_control_SOFC/Reformer  - SOFC System/SOFC Cell/Nernst’s Eq /MATLAB Function1 ==
  data: params input; V output; I input
function V = fcn(params, I)

A_esti =  params(1);
E0_esti =  params(2);
R_esti =  params(3);

m = 0.5355;
n = 0.0313;

I = abs(I);
V = E0_esti - I.*R_esti - A_esti*log(I) - m*exp(n*I);
